simulink model "preLookupTestGen28"  (R2017b)
settings: Solver=FixedStepDiscrete  StartTime=0.0  StopTime=10.0  RelTol=1e-3
undefined symbols (not defined in the file): Block_TestLib, enable_trigger
settings Model: Creator=ktrinh  LastModifiedBy=ktrinh
settings DebuggingCC: ParameterOverflowMsg=none

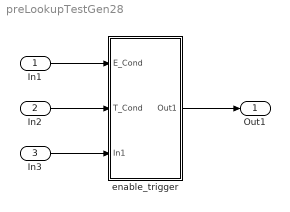
== system preLookupTestGen28 ==
  In1 : Inport
  In2 : Inport  Port=2
  In3 : Inport  Port=3
  enable_trigger : Subsystem  AncestorBlock=Block_TestLib/enable_trigger
  Out1 : Outport
  wires:
  In1/1 -> enable_trigger/1(E_Cond)
  In2/1 -> enable_trigger/2(T_Cond)
  In3/1 -> enable_trigger/3(In1)
  enable_trigger/1(Out1) -> Out1/1

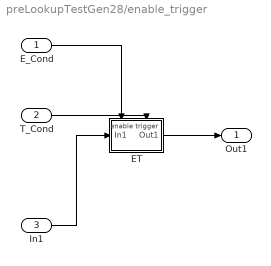
== system preLookupTestGen28/enable_trigger ==
  E_Cond : Inport  OutDataTypeStr=boolean
  T_Cond : Inport  Port=2  OutDataTypeStr=boolean
  In1 : Inport  Port=3
  ET : Subsystem  TreatAsAtomicUnit=on
  Out1 : Outport
  wires:
  T_Cond/1 -> ET/Trigger
  E_Cond/1 -> ET/Enable
  In1/1 -> ET/1(In1)
  ET/1(Out1) -> Out1/1

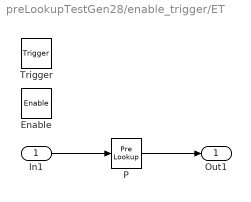
== system preLookupTestGen28/enable_trigger/ET ==
  In1 : Inport  OutDataTypeStr=double  PortDimensions=3
  Enable : EnablePort
  Trigger : TriggerPort  VariantControl=Variant
  P : PreLookup  InitFcn=|  BreakpointsData=[10:10:110]  BreakpointsSpecification=Even spacing  BreakpointsNumPoints=20  BreakpointsFirstPoint=54  BreakpointsSpacing=3  OutputSelection=Index and fraction as bus  IndexSearchMethod=Evenly spaced points  BreakpointDataTypeStr=int32  RndMeth=Ceiling  OutputBusDataTypeStr=Bus: kfBus
      | elems(1) = Simulink.BusElement;
      | elems(1).Name = 'Index';
      | elems(1).DataType = 'int8';
      | elems(2) = Simulink.BusElement;
      | elems(2).Name = 'Fraction';
      | elems(2).DataType = 'double';
      | kfBus = Simulink.Bus;
      | kfBus.Elements = elems;
      | clear elems;
      | assignin('base', 'kfBus', kfBus);
  Out1 : Outport
  wires:
  In1/1 -> P/1
  P/1 -> Out1/1
